simulink model "Maglev"  (R2024b)
settings: Solver=VariableStepAuto  StartTime=0.0  StopTime=2  RelTol=1e-3
libraries: fuzblock x2
settings Model: Creator=Dr.Red  LastModifiedBy=Dr.Red

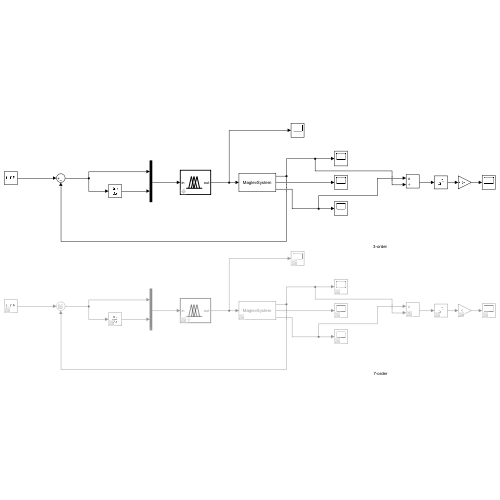
[thumbnail: Simulink's stored preview of the top-level diagram]
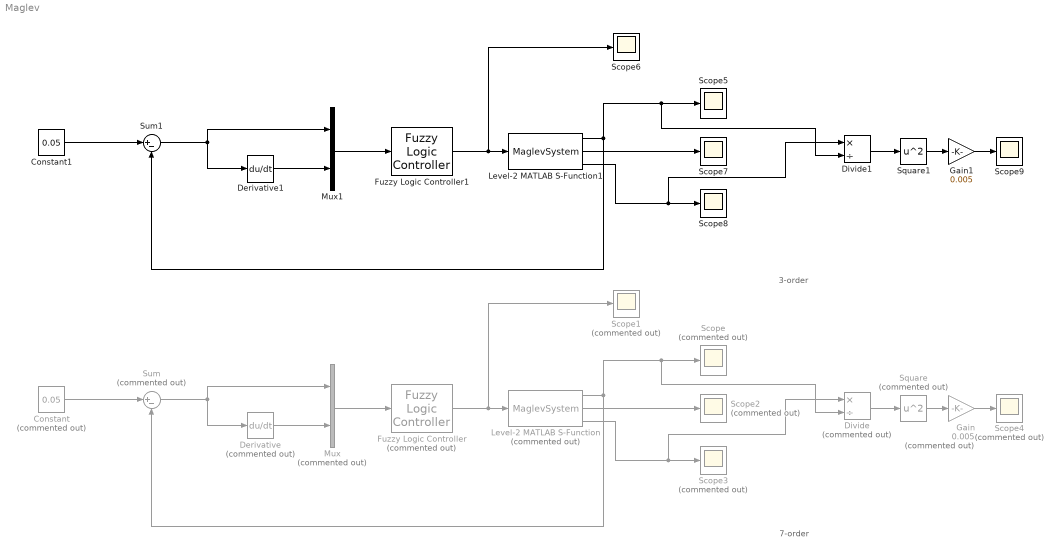
== system Maglev ==
  note: 7-order
  note: 3-order
  Constant : Constant  Commented=on  Value=0.05
  Constant1 : Constant  Value=0.05
  Derivative : Derivative  Commented=on
  Derivative1 : Derivative
  Divide : Product  Commented=on  Inputs=*/
  Divide1 : Product  Inputs=*/
  Fuzzy Logic Controller : fuzblock/Fuzzy Logic  Controller  Commented=on  FIS='fuzzy.fis'  OutputSampleNumber=101  DataType=double  FuzzifiedInputs=off  RuleFiringStrengths=off  RuleOutputs=off  AggregatedOutputs=off  SimulateUsing=Interpreted execution  OutOfRangeInputValueMessage=warning  NoRuleFiredMessage=warning  EmptyOutputFuzzySetMessage=warning
  Fuzzy Logic Controller1 : fuzblock/Fuzzy Logic  Controller  FIS='fuzzy1.fis'  OutputSampleNumber=101  DataType=double  FuzzifiedInputs=off  RuleFiringStrengths=off  RuleOutputs=off  AggregatedOutputs=off  SimulateUsing=Interpreted execution  OutOfRangeInputValueMessage=warning  NoRuleFiredMessage=warning  EmptyOutputFuzzySetMessage=warning
  Gain : Gain  Commented=on  Gain=0.005
  Gain1 : Gain  Gain=0.005
  Level-2 MATLAB S-Function : M-S-Function  Commented=on  FunctionName=MaglevSystem  Parameters=0.03,0,0
  Level-2 MATLAB S-Function1 : M-S-Function  FunctionName=MaglevSystem  Parameters=0.03,0,0
  Mux : Mux  Commented=on  Inputs=2
  Mux1 : Mux  Inputs=2
  Scope{,1..4} (5 alike) : Scope  Commented=on
  Scope{5..9} (5 alike) : Scope
  Square : Math  Commented=on  Operator=square
  Square1 : Math  Operator=square
  Sum : Sum  Commented=on  Inputs=|+-
  Sum1 : Sum  Inputs=|+-
  wires:
  Constant/1 -> Sum/1
  Level-2 MATLAB S-Function/1 -> Divide/2, Scope/1, Sum/2
  Level-2 MATLAB S-Function/2 -> Scope2/1
  Level-2 MATLAB S-Function/3 -> Divide/1, Scope3/1
  Sum/1 -> Mux/1, Derivative/1
  Mux/1 -> Fuzzy Logic Controller/1
  Derivative/1 -> Mux/2
  Divide/1 -> Square/1
  Square/1 -> Gain/1
  Gain/1 -> Scope4/1
  Fuzzy Logic Controller/1 -> Level-2 MATLAB S-Function/1, Scope1/1
  Gain1/1 -> Scope9/1
  Square1/1 -> Gain1/1
  Mux1/1 -> Fuzzy Logic Controller1/1
  Constant1/1 -> Sum1/1
  Derivative1/1 -> Mux1/2
  Fuzzy Logic Controller1/1 -> Level-2 MATLAB S-Function1/1, Scope6/1
  Level-2 MATLAB S-Function1/3 -> Divide1/1, Scope8/1
  Level-2 MATLAB S-Function1/2 -> Scope7/1
  Sum1/1 -> Mux1/1, Derivative1/1
  Divide1/1 -> Square1/1
  Level-2 MATLAB S-Function1/1 -> Divide1/2, Scope5/1, Sum1/2
